simulink model "filter_4"  (R2020a)
settings: Solver=FixedStepDiscrete  StartTime=0.0  StopTime=10.0  RelTol=1e-3
settings Model: Creator=Prateek  LastModifiedBy=Prateek
settings DataIOCC: SaveOutput=off  SaveTime=off

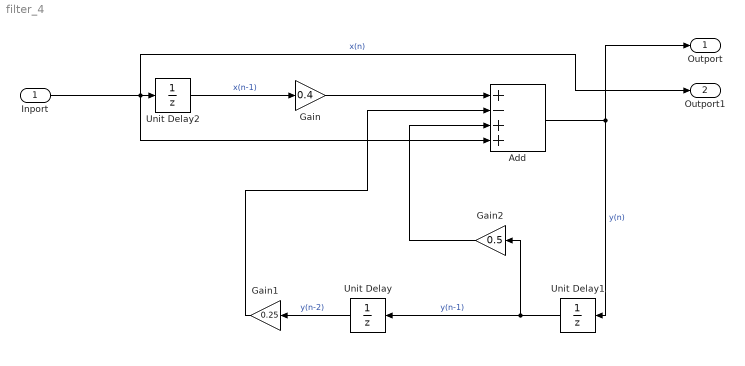
== system filter_4 ==
  Inport : Inport  OutDataTypeStr=double  PortDimensions=1  SampleTime=0
  Add : Sum  Inputs=+-++
  Gain : Gain  Gain=0.4
  Gain1 : Gain  Gain=0.25
  Gain2 : Gain  Gain=0.5
  Unit Delay : UnitDelay  SampleTime=-1  HasFrameUpgradeWarning=on
  Unit Delay1 : UnitDelay  SampleTime=-1  HasFrameUpgradeWarning=on
  Unit Delay2 : UnitDelay  SampleTime=-1  HasFrameUpgradeWarning=on
  Outport : Outport  OutDataTypeStr=double  PortDimensions=1  SampleTime=0
  Outport1 : Outport  Port=2  OutDataTypeStr=double  PortDimensions=1  SampleTime=0
  wires:
  Inport/1 -> Add/4, Unit Delay2/1, Outport1/1  "x(n)"
  Gain1/1 -> Add/2
  Unit Delay/1 -> Gain1/1  "y(n-2)"
  Gain/1 -> Add/1
  Unit Delay2/1 -> Gain/1  "x(n-1)"
  Add/1 -> Unit Delay1/1, Outport/1  "y(n)"
  Unit Delay1/1 -> Gain2/1, Unit Delay/1  "y(n-1)"
  Gain2/1 -> Add/3
